simulink model "sytem_m2"  (R2017a)
settings: Solver=FixedStepDiscrete  StartTime=0.0  StopTime=500  RelTol=1e-3
libraries: simulink x1
settings Model: Creator=dsmv8  LastModifiedBy=dsmv8
settings OptimizationCC: DefaultUnderspecifiedDataType=single

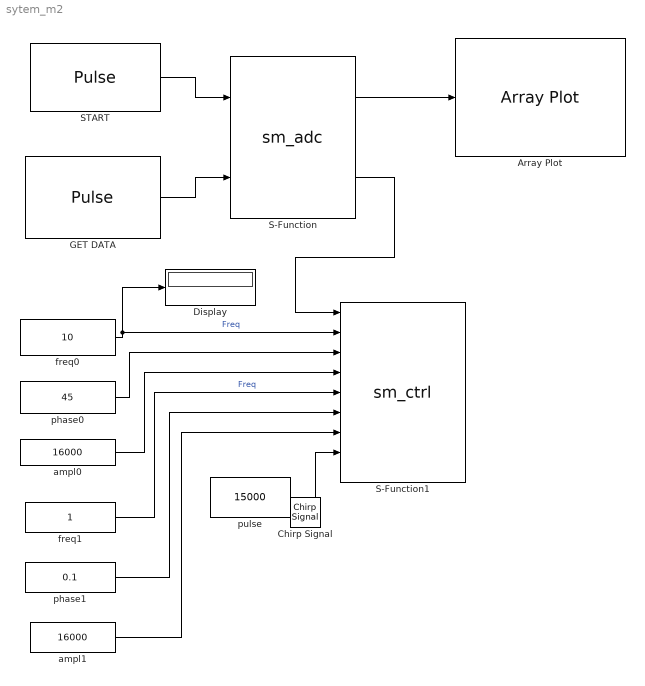
== system sytem_m2 ==
  Array Plot : ArrayPlot
  Display : Display
  "GET DATA " : DiscretePulseGenerator  PulseType=Time based  Amplitude=512  Period=0.1  PulseWidth=10  SampleTime=0.0001
  S-Function : S-Function  FunctionName=sm_adc  Parameters='SimulinkAdc' 1024  SFunctionDeploymentMode=off  EnableBusSupport=off
  S-Function1 : S-Function  FunctionName=sm_ctrl  Parameters='SimulinkCtrl'  SFunctionDeploymentMode=off  EnableBusSupport=off
  START : DiscretePulseGenerator  PulseType=Time based  Amplitude=400  Period=0.1  PulseWidth=10  PhaseDelay=0.08  SampleTime=0.0001
  "ampl0 " : Constant  Value=16000
  ampl1 : Constant  Value=16000
  freq0 : Constant  Value=10
  freq1 : Constant
  phase0 : Constant  Value=45
  phase1 : Constant  Value=0.1
  pulse : Constant  Value=15000
  Chirp Signal : simulink/Sources/Chirp Signal  IOType=siggen  f1=0.1  T=100  f2=1
  wires:
  S-Function/1 -> Array Plot/1
  freq0/1 -> S-Function1/2, Display/1  "Freq"
  "GET DATA "/1 -> S-Function/2
  phase0/1 -> S-Function1/3
  "ampl0 "/1 -> S-Function1/4
  freq1/1 -> S-Function1/5  "Freq"
  phase1/1 -> S-Function1/6
  ampl1/1 -> S-Function1/7
  pulse/1 -> S-Function1/8
  START/1 -> S-Function/1
  S-Function/2 -> S-Function1/1
